simulink model "inverter_model"  (R2016a)
settings: Solver=VariableStepAuto  StartTime=0.0  StopTime=10e-2  RelTol=1e-3
libraries: powerlib x15, powerlib_meascontrol x1
settings Model: Creator=Doga  LastModifiedBy=Doga

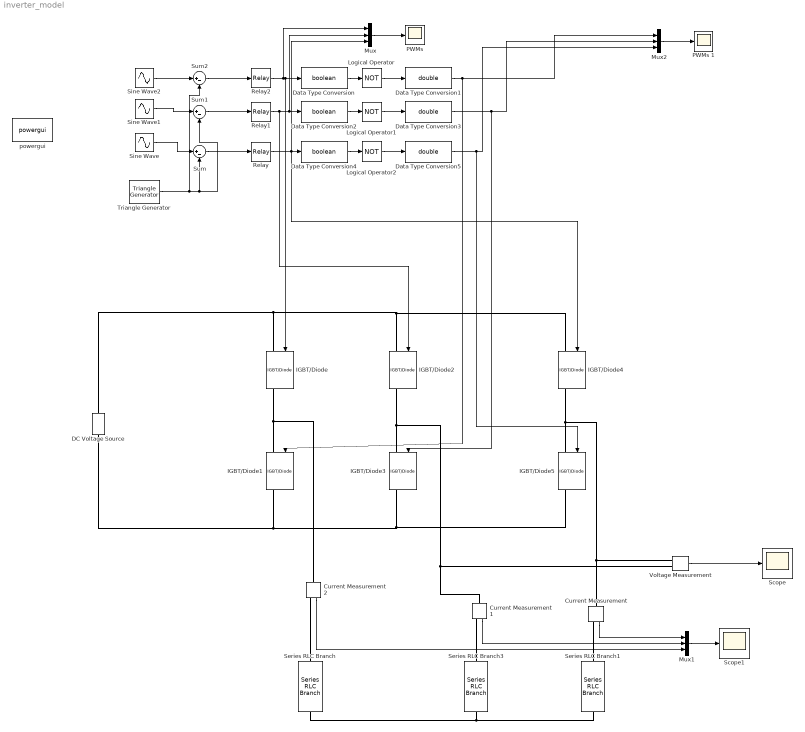
== system inverter_model ==
  Current Measurement : powerlib/Measurements/Current Measurement  PhasorSimulation=off  OutputType=Complex  PSBequivalent=0
  Current Measurement1 : powerlib/Measurements/Current Measurement  PhasorSimulation=off  OutputType=Complex  PSBequivalent=0
  Current Measurement2 : powerlib/Measurements/Current Measurement  PhasorSimulation=off  OutputType=Complex  PSBequivalent=0
  DC Voltage Source : powerlib/Electrical Sources/DC Voltage Source  Amplitude=400  Measurements=None
  Data Type Conversion : DataTypeConversion  OutDataTypeStr=boolean
  Data Type Conversion1 : DataTypeConversion  OutDataTypeStr=double
  Data Type Conversion2 : DataTypeConversion  OutDataTypeStr=boolean
  Data Type Conversion3 : DataTypeConversion  OutDataTypeStr=double
  Data Type Conversion4 : DataTypeConversion  OutDataTypeStr=boolean
  Data Type Conversion5 : DataTypeConversion  OutDataTypeStr=double
  IGBT/Diode{,1..5} (6 alike) : powerlib/Power Electronics/IGBT//Diode  Ron=1e-3  Rs=1e5  Cs=inf  Measurements=on
  Logical Operator : Logic  Operator=NOT  AllPortsSameDT=off  OutDataTypeStr=boolean
  Logical Operator1 : Logic  Operator=NOT  AllPortsSameDT=off  OutDataTypeStr=boolean
  Logical Operator2 : Logic  Operator=NOT  AllPortsSameDT=off  OutDataTypeStr=boolean
  Mux : Mux  Inputs=3
  Mux1 : Mux  Inputs=3
  Mux2 : Mux  Inputs=3
  "PWMs " : Scope
  PWMs 1 : Scope
  Relay : Relay
  Relay1 : Relay
  Relay2 : Relay
  Scope : Scope
  Scope1 : Scope
  Series RLC Branch : powerlib/Elements/Series RLC Branch  LConnTagsString=__new0  RConnTagsString=__new0  BranchType=RL  Resistance=16.25  Inductance=0.0245  SetiL0=off  InitialCurrent=0  Capacitance=1e-6  Setx0=off  InitialVoltage=0  Measurements=None
  Series RLC Branch1 : powerlib/Elements/Series RLC Branch  LConnTagsString=__new0  RConnTagsString=__new0  BranchType=RL  Resistance=16.25  Inductance=0.0245  SetiL0=off  InitialCurrent=0  Capacitance=1e-6  Setx0=off  InitialVoltage=0  Measurements=None
  Series RLC Branch3 : powerlib/Elements/Series RLC Branch  LConnTagsString=__new0  RConnTagsString=__new0  BranchType=RL  Resistance=16.25  Inductance=0.0245  SetiL0=off  InitialCurrent=0  Capacitance=1e-6  Setx0=off  InitialVoltage=0  Measurements=None
  Sine Wave : Sin  Amplitude=200/(400*0.612)  Frequency=314  SampleTime=0
  Sine Wave1 : Sin  Amplitude=200/(400*0.612)  Frequency=314  Phase=4*pi/3  SampleTime=0
  Sine Wave2 : Sin  Amplitude=200/(400*0.612)  Frequency=314  Phase=8*pi/3  SampleTime=0
  Sum : Sum  Inputs=|+-
  Sum1 : Sum  Inputs=|+-
  Sum2 : Sum  Inputs=|+-
  Triangle Generator : powerlib_meascontrol/Pulse & Signal Generators/Triangle Generator  Freq=1000  Phase=90  Ts=0
  Voltage Measurement : powerlib/Measurements/Voltage Measurement  PhasorSimulation=off  OutputType=Complex  PSBequivalent=0
  powergui : powerlib/powergui  Priority=1  SimulationMode=Continuous  SolverType=Tustin/Backward Euler (TBE)  SampleTime=50e-6  frequency=60  SPID=off  DisableSnubberDevices=off  DisableRonSwitches=off  DisableVfSwitches=off  SwTol=0  DisplayEquations=off  Interpol=off  ExternalGateDelay=off  methode=off  Ts=10  FunctionMessages=off  echomessages=off  HookPort=off  EnableUseOfTLC=off  x0status=blocks  frequencyindice=0  Pbase=100e6  ErrMax=1e-4  Iterations=50  UnitsV=kV  UnitsW=MW  buscounter=0  RestoreLinks=warning  ResistiveCurrentMeasurement=off  Frange=[0:2:500]  Ylog=off  Xlog=on  ShowGrid=off  save=off  variable=ZData  structure=0  ZoomFFT=off  StartTime=0.0  cycles=1  DisplayStyle=1  fundamental=60  FreqAxis=off  MaxFrequency=1000  frequencyindicesteady=1  RmsSteady=1  display=off
  wires:
  Triangle Generator/1 -> Sum1/2, Sum/2, Sum2/2
  Sine Wave/1 -> Sum/1
  Sum/1 -> Relay/1
  Sine Wave1/1 -> Sum1/1
  Sine Wave2/1 -> Sum2/1
  Sum2/1 -> Relay2/1
  Sum1/1 -> Relay1/1
  Mux/1 -> "PWMs "/1
  Relay2/1 -> IGBT/Diode/1, Data Type Conversion/1, Mux/1
  Data Type Conversion/1 -> Logical Operator/1
  Logical Operator/1 -> Data Type Conversion1/1
  Relay1/1 -> IGBT/Diode2/1, Mux/2, Data Type Conversion2/1
  Data Type Conversion2/1 -> Logical Operator1/1
  Logical Operator1/1 -> Data Type Conversion3/1
  Relay/1 -> IGBT/Diode4/1, Mux/3, Data Type Conversion4/1
  Data Type Conversion4/1 -> Logical Operator2/1
  Logical Operator2/1 -> Data Type Conversion5/1
  Voltage Measurement/1 -> Scope/1
  Current Measurement/1 -> Mux1/1
  Current Measurement1/1 -> Mux1/2
  Current Measurement2/1 -> Mux1/3
  Mux1/1 -> Scope1/1
  Mux2/1 -> PWMs 1/1
  Data Type Conversion1/1 -> IGBT/Diode1/1, Mux2/1
  Data Type Conversion3/1 -> Mux2/2, IGBT/Diode3/1
  Data Type Conversion5/1 -> IGBT/Diode5/1, Mux2/3
  connections:
  IGBT/Diode2/RConn1 -- Voltage Measurement/LConn2 -- Current Measurement1/LConn1 -- IGBT/Diode3/LConn1
  DC Voltage Source/RConn1 -- IGBT/Diode4/LConn1 -- IGBT/Diode2/LConn1 -- IGBT/Diode/LConn1
  DC Voltage Source/LConn1 -- IGBT/Diode5/RConn1 -- IGBT/Diode3/RConn1 -- IGBT/Diode1/RConn1
  IGBT/Diode/RConn1 -- Current Measurement2/LConn1 -- IGBT/Diode1/LConn1
  Series RLC Branch3/RConn1 -- Series RLC Branch1/RConn1 -- Series RLC Branch/RConn1
  IGBT/Diode5/LConn1 -- Voltage Measurement/LConn1 -- Current Measurement/LConn1 -- IGBT/Diode4/RConn1
  Series RLC Branch1/LConn1 -- Current Measurement/RConn1
  Series RLC Branch3/LConn1 -- Current Measurement1/RConn1
  Current Measurement2/RConn1 -- Series RLC Branch/LConn1
